simulink model "OPC_UA_Test"  (R2024b)
settings: Solver=FixedStepDiscrete  StartTime=0.0  StopTime=inf  FixedStep=0.01  MaxStep=0.001  RelTol=1e-3
libraries: opcualib x1, sldrtlib x1
settings Model: Creator=Green Crane Testbed  LastModifiedBy=Green Crane Testbed

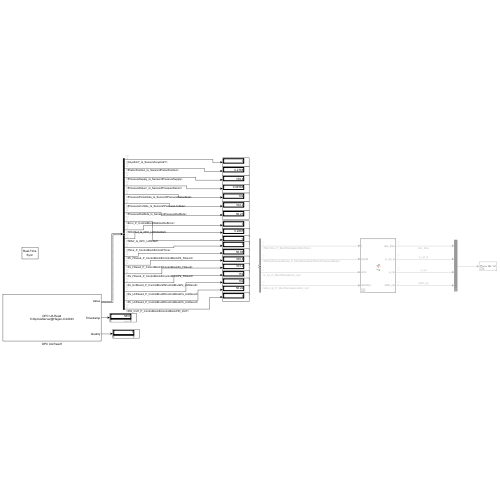
[thumbnail: Simulink's stored preview of the top-level diagram]
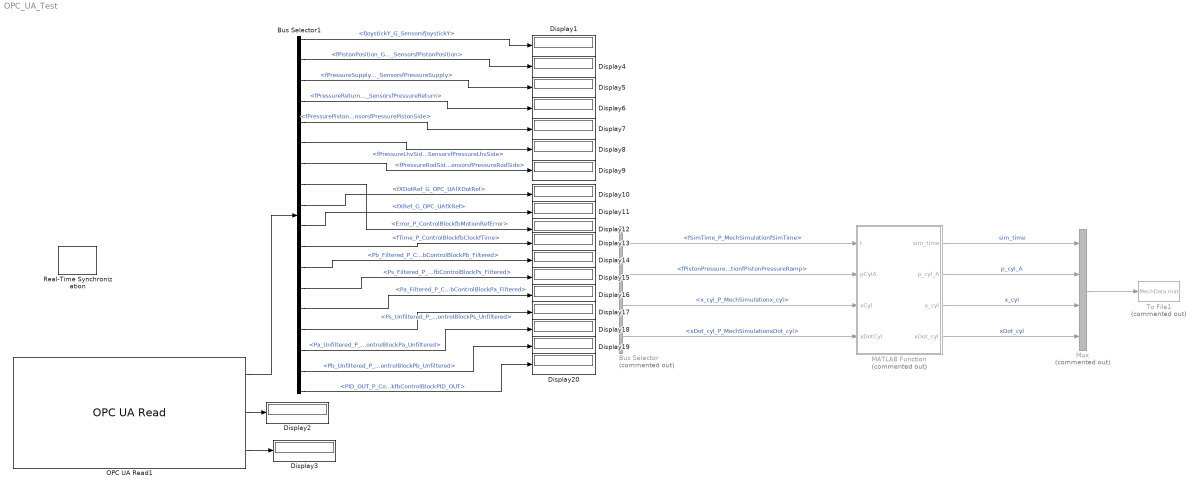
== system OPC_UA_Test ==
  Bus Selector : BusSelector  Commented=on  OutputSignals=fSimTime_P_MechSimulationfSimTime,fPistonPressureRamp_P_MechSimulationfPistonPressureRamp,x_cyl_P_MechSimulationx_cyl,xDot_cyl_P_MechSimulationxDot_cyl
  Bus Selector1 : BusSelector  OutputSignals=fJoystickY_G_SensorsfJoystickY,fPistonPosition_G_SensorsfPistonPosition,fPressureSupply_G_SensorsfPressureSupply,fPressureReturn_G_SensorsfPressureReturn,fPressurePistonSide_G_SensorsfPressurePistonSide,fPressureLhvSide_G_SensorsfPressureLhvSide,fPressureRodSide_G_SensorsfPressureRodSide,Error_P_ControlBlockfbMotionRefError,fXDotRef_G_OPC_UAfXDotRef,fXRef_G_OPC_UAfXRef,fTime_P_ControlBlockfbClockfTime,Pb_Filtered_P_ControlBlockfbControlBlockPb_Filtered,Ps_Filtered_P_ControlBlockfbControlBlockPs_Filtered,Pa_Filtered_P_ControlBlockfbControlBlockPa_Filtered,Ps_Unfiltered_P_ControlBlockfbControlBlockPs_Unfiltered,Pa_Unfiltered_P_ControlBlockfbControlBlockPa_Unfiltered,Pb_Unfiltered_P_ControlBlockfbControlBlockPb_Unfiltered,PID_OUT_P_ControlBlockfbControlBlockPID_OUT
  Display{1..20} (20 alike) : Display
  MATLAB Function : MATLAB Function  Commented=on  TreatAsAtomicUnit=on
  Mux : Mux  Commented=on
  OPC UA Read1 : opcualib/OPC UA Read  SelectedServer=TcOpcUaServer@Hagen-CX2043  ServerList=TcOpcUaServer@Hagen-CX2043  NodeList={ '1', 'fJoystickY', '4', 'G_Sensors.fJoystickY', '0'; '2', 'fPistonPosition', '4', 'G_Sensors.fPistonPosition', '0'; '3', 'fPressureSupply', '4', 'G_Sensors.fPressureSupply', '0'; '4', 'fPressureReturn', '4', 'G_Sensors.fPressureReturn', '0'; '5', 'fPressurePistonSide', '4', 'G_Sensors.fPressurePistonSide', '0'; '6', 'fPressureLhvSide', '4', 'G_Sensors.fPressureLhvSide', '0'; '7', 'fPressureRodSide', '4', 'G_Sensors.fPressureRodSide', '0'; '8', 'fPositionReference_m', '4', 'P_ControlBlock.fbMotionRef.fPositionReference_m', '0'; '9', 'fVelocityReference_ms', '4', 'P_ControlBlock.fbMotionRef.fVelocityReference_ms', '0'; '10', 'Error', '4', 'P_ControlBlock.fbMotionRef.Error', '0'; '11', 'fTime', '4', 'P_ControlBlock.fbClock.fTime', '0'; '12', 'Pb_Filtered', '4', 'P_ControlBlock.fbControlBlock.Pb_Filtered', '0'; '13', 'Ps_Filtered', '4', 'P_ControlBlock.fbControlBlock.Ps_Filtered', '0'; '14', 'Pa_Filtered', '4', 'P_ControlBlock.fbControlBlock.Pa_Filtered', '0'; '15', 'Ps_Unfiltered', '4', 'P_ControlBlock.fbControlBlock.Ps_Unfiltered', '0'; '16', 'Pa_Unfiltered', '4', 'P_ControlBlock.fbControlBlock.Pa_Unfiltered', '0'; '17', 'Pb_Unfiltered', '4', 'P_ControlBlock.fbControlBlock.Pb_Unfiltered', '0'; '18', 'PID_OUT', '4', 'P_ControlBlock.fbControlBlock.PID_OUT', '0'; '19', 'fXRef', '4', 'G_OPC_UA.fXRef', '0'; '20', 'fXDotRef', '4', 'G_OPC_UA.fXDotRef', '0' }  ShowQualityPort=on  ShowTimestampPort=on  ShowTimestampPortAs=Seconds since start  SampleTime=-1
  Real-Time Synchronization : sldrtlib/Real-Time Synchronization  SampleTime=-1  MaxMissedTicks=1000000000000  ShowMissedTicks=off  YieldWhenWaiting=off
  To File1 : ToFile  Commented=on  Filename=MechData.mat  SaveFormat=Timeseries
  wires:
  Bus Selector/1 -> MATLAB Function/1(t)  "<fSimTime_P_MechSimulationfSimTime>"
  Bus Selector/2 -> MATLAB Function/2(pCylA)  "<fPistonPressureRamp_P_MechSimulationfPistonPressureRamp>"
  Bus Selector/3 -> MATLAB Function/3(xCyl)  "<x_cyl_P_MechSimulationx_cyl>"
  Bus Selector/4 -> MATLAB Function/4(xDotCyl)  "<xDot_cyl_P_MechSimulationxDot_cyl>"
  MATLAB Function/1(sim_time) -> Mux/1  "sim_time"
  MATLAB Function/2(p_cyl_A) -> Mux/2  "p_cyl_A"
  MATLAB Function/3(x_cyl) -> Mux/3  "x_cyl"
  MATLAB Function/4(xDot_cyl) -> Mux/4  "xDot_cyl"
  Mux/1 -> To File1/1
  OPC UA Read1/1 -> Bus Selector1/1
  OPC UA Read1/3 -> Display3/1
  OPC UA Read1/2 -> Display2/1
  Bus Selector1/1 -> Display1/1  "<fJoystickY_G_SensorsfJoystickY>"
  Bus Selector1/2 -> Display4/1  "<fPistonPosition_G_SensorsfPistonPosition>"
  Bus Selector1/3 -> Display5/1  "<fPressureSupply_G_SensorsfPressureSupply>"
  Bus Selector1/4 -> Display6/1  "<fPressureReturn_G_SensorsfPressureReturn>"
  Bus Selector1/5 -> Display7/1  "<fPressurePistonSide_G_SensorsfPressurePistonSide>"
  Bus Selector1/6 -> Display8/1  "<fPressureLhvSide_G_SensorsfPressureLhvSide>"
  Bus Selector1/7 -> Display9/1  "<fPressureRodSide_G_SensorsfPressureRodSide>"
  Bus Selector1/8 -> Display12/1  "<Error_P_ControlBlockfbMotionRefError>"
  Bus Selector1/11 -> Display13/1  "<fTime_P_ControlBlockfbClockfTime>"
  Bus Selector1/12 -> Display14/1  "<Pb_Filtered_P_ControlBlockfbControlBlockPb_Filtered>"
  Bus Selector1/13 -> Display15/1  "<Ps_Filtered_P_ControlBlockfbControlBlockPs_Filtered>"
  Bus Selector1/14 -> Display16/1  "<Pa_Filtered_P_ControlBlockfbControlBlockPa_Filtered>"
  Bus Selector1/15 -> Display17/1  "<Ps_Unfiltered_P_ControlBlockfbControlBlockPs_Unfiltered>"
  Bus Selector1/16 -> Display18/1  "<Pa_Unfiltered_P_ControlBlockfbControlBlockPa_Unfiltered>"
  Bus Selector1/17 -> Display19/1  "<Pb_Unfiltered_P_ControlBlockfbControlBlockPb_Unfiltered>"
  Bus Selector1/18 -> Display20/1  "<PID_OUT_P_ControlBlockfbControlBlockPID_OUT>"
  Bus Selector1/9 -> Display10/1  "<fXDotRef_G_OPC_UAfXDotRef>"
  Bus Selector1/10 -> Display11/1  "<fXRef_G_OPC_UAfXRef>"

== matlab function OPC_UA_Test/MATLAB Function ==
  data: t input; sim_time output; p_cyl_A output; x_cyl output; xDot_cyl output; pCylA input; xCyl input; xDotCyl input
function [sim_time, p_cyl_A, x_cyl, xDot_cyl]   = fcn(t, pCylA, xCyl, xDotCyl)
if t >= 0.0 && t < 10.0
     sim_time = t;
     p_cyl_A = pCylA;
     x_cyl = xCyl;
     xDot_cyl = xDotCyl;
elseif t >= 10.0
     sim_time = 10.0;
     p_cyl_A = pCylA;
     x_cyl = xCyl;
     xDot_cyl = xDotCyl;
else
     sim_time = 0.0;
     p_cyl_A = 0.0;
     x_cyl = 0.0;
     xDot_cyl = 0.0;
end
